simulink model "aero_vibrati"  (Simulink 6.0)
settings: Solver=ode5  SolverMode=SingleTasking  StartTime=0.0  StopTime=20.0  FixedStep=.01  RelTol=1e-3  AbsTol=1e-6
values from neighbouring files (symbols this model uses):
  omega = 2*pi*5    (= 31.4159265359)    [aero_pointer_tracker.m]
  zeta = .01    (= 0.01)    [aero_pointer_tracker.m]
settings Model: Creator=The MathWorks Inc.  LastModifiedBy=batserve  ExtModeTrigMode=oneshot  ExtModeArmWhenConnect=off  ExtModeAutoUpdateStatusClock=off
settings DataIOCC: LimitDataPoints=off  TimeSaveName=Time
settings OptimizationCC: BlockReduction=off  BooleanDataType=off
settings DebuggingCC: CheckExecutionContextPreStartOutputMsg=on  CheckExecutionContextRuntimeOutputMsg=on  SolverPrmCheckMsg=none
settings HardwareCC: TargetUnknown=on

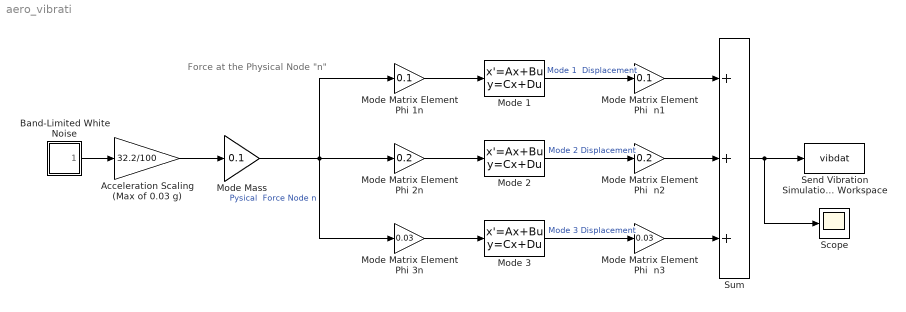
== system aero_vibrati ==
  note: Force  at the Physical
      | Node "n"
  Acceleration Scaling (Max of 0.03 g) : Gain  Gain=32.2/100  SaturateOnIntegerOverflow=on
  Band-Limited White Noise : Subsystem  PropExecContextAcrossSSBoundary=on  mask(Continuous White Noise.){Cov=[0.1], Ts=0.01, seed=rand}
      mask prompts: Cov "Noise Power:"; Ts "Sample time:"
      mask help: White noise for continuous (s-domain) systems. Band-limited using zero-order-hold.
      mask init:
      | r = rand(1,12); r2 = [r(1),r;r,r(12)]; t =[1:13;1:13];
      mask Help: Implemented using white noise into Zero-Order Hold block. The seed and power can be vectors of the same length to produce a vector of white noise sources. For faster simulation, set sample time to the highest value possible but in accordance with the fastest dynamics of system.
      mask Display: plot(t(:),r2(:))
  Mode Mass : Gain  Gain=0.1  SaturateOnIntegerOverflow=on
  Mode 1 : StateSpace  A=[0 1;-omega^2 -2*zeta*omega]  B=[0 omega^2]'  C=[1 0]  D=0
  Mode 2 : StateSpace  A=[0 1;-(2*omega)^2 -2*zeta*2*omega]  B=[0 omega^2]'  C=[1 0]  D=0
  Mode 3 : StateSpace  A=[0 1;-(3*omega)^2 -2*zeta*3*omega]  B=[0 omega^2]'  C=[1 0]  D=0
  Mode Matrix Element Phi  n1 : Gain  Gain=0.1  SaturateOnIntegerOverflow=on
  Mode Matrix Element Phi  n2 : Gain  Gain=0.2  SaturateOnIntegerOverflow=on
  Mode Matrix Element Phi  n3 : Gain  Gain=0.03  SaturateOnIntegerOverflow=on
  Mode Matrix Element Phi 1n : Gain  Gain=0.1  SaturateOnIntegerOverflow=on
  Mode Matrix Element Phi 2n : Gain  Gain=0.2  SaturateOnIntegerOverflow=on
  Mode Matrix Element Phi 3n : Gain  Gain=0.03  SaturateOnIntegerOverflow=on
  Scope : Scope
      settings: TickLabels=on  YMin=-0.02  YMax=0.02  DataFormat=Array
  Send Vibration Simulation to Workspace : ToWorkspace  VariableName=vibdat  SampleTime=0.01  SaveFormat=Array
  Sum : Sum  Inputs=+++  SaturateOnIntegerOverflow=on  InputSameDT=on
  wires:
  Band-Limited White Noise/1(Out_1) -> Acceleration Scaling (Max of 0.03 g)/1
  Acceleration Scaling (Max of 0.03 g)/1 -> Mode Mass/1
  Mode Mass/1 -> Mode Matrix Element Phi 2n/1, Mode Matrix Element Phi 1n/1, Mode Matrix Element Phi 3n/1  "Pysical  Force Node n"
  Mode Matrix Element Phi 2n/1 -> Mode 2/1
  Mode Matrix Element Phi 1n/1 -> Mode 1/1
  Mode Matrix Element Phi  n2/1 -> Sum/2
  Mode Matrix Element Phi  n1/1 -> Sum/1
  Mode 2/1 -> Mode Matrix Element Phi  n2/1  "Mode 2 Displacement"
  Mode 1/1 -> Mode Matrix Element Phi  n1/1  "Mode 1  Displacement"
  Mode Matrix Element Phi 3n/1 -> Mode 3/1
  Mode Matrix Element Phi  n3/1 -> Sum/3
  Mode 3/1 -> Mode Matrix Element Phi  n3/1  "Mode 3 Displacement"
  Sum/1 -> Send Vibration Simulation to Workspace/1, Scope/1

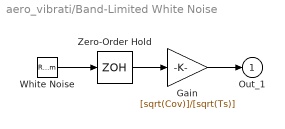
== system aero_vibrati/Band-Limited White Noise ==
  Gain : Gain  Gain=[sqrt(Cov)]/[sqrt(Ts)]  SaturateOnIntegerOverflow=on
  White Noise : RandomNumber  Seed=seed  SampleTime=0
  Zero-Order Hold : ZeroOrderHold  SampleTime=Ts
  Out_1 : Outport  InitialOutput=0
  wires:
  Zero-Order Hold/1 -> Gain/1
  Gain/1 -> Out_1/1
  White Noise/1 -> Zero-Order Hold/1
